simulink model "HW1_Q1"  (R2018a)
settings: Solver=VariableStepAuto  StartTime=0.0  StopTime=50.0  FixedStep=0.01  RelTol=1e-3
settings Model: Creator=labuser  LastModifiedBy=Halil Temurtaş
settings CodeAppCC: StateflowObjectComments=on

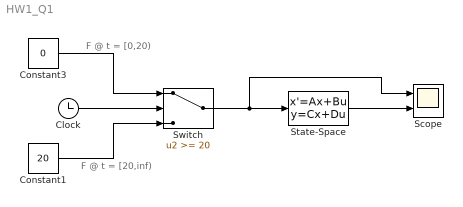
== system HW1_Q1 ==
  note: F @ t = [0,20)
  note: F @ t = [20,inf)
  Clock : Clock
  Constant1 : Constant  Value=20
  Constant3 : Constant  Value=0
  Scope : Scope  NumInputPorts=2
  State-Space : StateSpace  A=[0 1; -1 -0.2]  B=[0 ; 1]  C=[1 0]  D=[0]  InitialCondition=0  ContinuousStateAttributes={'position','velocity'}
  Switch : Switch  Threshold=20
  wires:
  State-Space/1 -> Scope/2
  Clock/1 -> Switch/2
  Constant3/1 -> Switch/1
  Constant1/1 -> Switch/3
  Switch/1 -> Scope/1, State-Space/1
